simulink model "Electron_Rocket_test_failed"  (R2023a)
settings: Solver=ode45  StartTime=0.0  StopTime=5000  RelTol=1e-6
undefined symbols (not defined in the file or in its folder): Earth, WGS84
libraries: simulink x3, aerolibadyn x1, aerolibatmos2 x1, slpidlib x1, simulink_extras x1, aerolib6dof2 x1
settings Model: Creator=User  LastModifiedBy=User

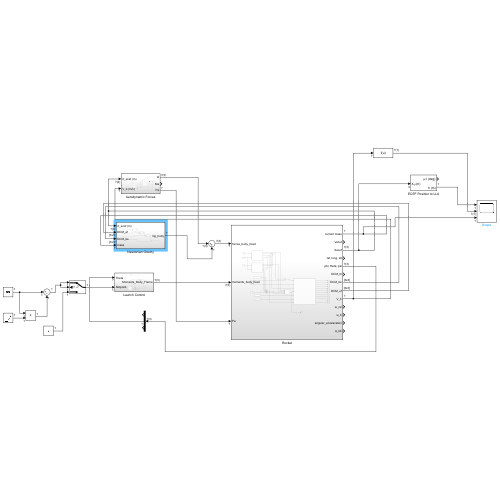
[thumbnail: Simulink's stored preview of the top-level diagram]
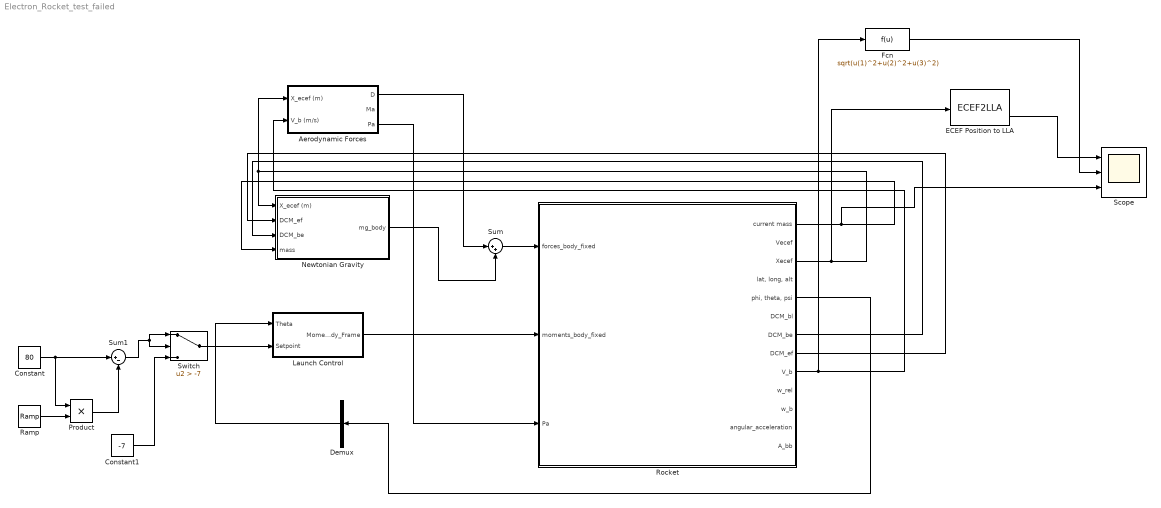
== system Electron_Rocket_test_failed ==
  Aerodynamic Forces : Subsystem
  Constant : Constant  Value=80
  Constant1 : Constant  Value=-7
  Demux : Demux  Outputs=3
  ECEF Position to LLA : ECEF2LLA
  Fcn : Fcn  Expr=sqrt(u(1)^2+u(2)^2+u(3)^2)
  Launch Control : Subsystem
  Newtonian Gravity : Subsystem
  Product : Product
  Ramp : simulink/Sources/Ramp  slope=0.0085  start=15  InitialOutput=0
  Rocket : Subsystem
  Scope : Scope  NumInputPorts=3
  Sum : Sum  Inputs=|++
  Sum1 : Sum  Inputs=|+-
  Switch : Switch  Criteria=u2 > Threshold  Threshold=-7  SaturateOnIntegerOverflow=off  InputSameDT=off
  wires:
  Rocket/3(Xecef) -> ECEF Position to LLA/1, Aerodynamic Forces/1(X_ecef (m)), Newtonian Gravity/1(X_ecef (m))
  Rocket/9(V_b) -> Fcn/1, Aerodynamic Forces/2(V_b (m/s))
  Rocket/1(current mass) -> Scope/3, Newtonian Gravity/4(mass)
  Rocket/7(DCM_be) -> Newtonian Gravity/3(DCM_be)
  Rocket/8(DCM_ef) -> Newtonian Gravity/2(DCM_ef)
  Aerodynamic Forces/1(D) -> Sum/1
  Newtonian Gravity/1(mg_body) -> Sum/2
  Sum/1 -> Rocket/1(forces_body_fixed)
  Aerodynamic Forces/3(Pa) -> Rocket/3(Pa)
  Launch Control/1(Moments_Body_Frame) -> Rocket/2(moments_body_fixed)
  Rocket/5("phi, theta, psi") -> Demux/1
  Demux/2 -> Launch Control/1(Theta)
  Constant/1 -> Sum1/1, Product/1
  Ramp/1 -> Product/2
  Sum1/1 -> Switch/1, Switch/2
  Switch/1 -> Launch Control/2(Setpoint)
  Constant1/1 -> Switch/3
  Product/1 -> Sum1/2
  ECEF Position to LLA/2 -> Scope/1
  Fcn/1 -> Scope/2

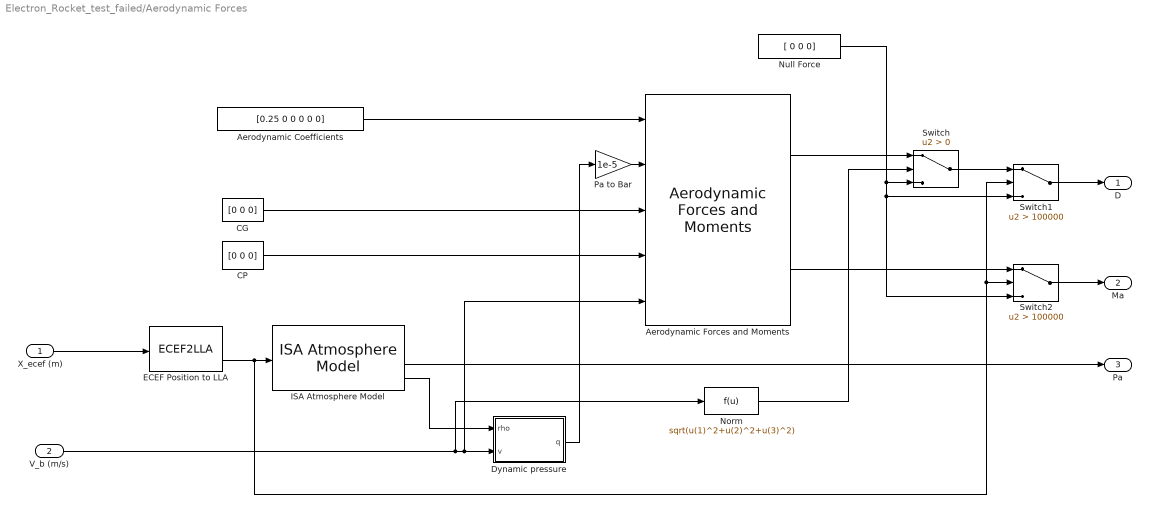
== system Electron_Rocket_test_failed/Aerodynamic Forces ==
  X_ecef (m) : Inport
  V_b (m/s) : Inport  Port=2
  "Aerodynamic Forces and Moments " : aerolibadyn/Aerodynamic Forces and Moments   inputAxes=Wind  outputForceAxes=Body  outputMomentAxes=Body  S=0.78  b=1  cbar=17
  Aerodynamic Coefficients : Constant  Value=[0.25 0 0 0 0 0]
  CG : Constant  Value=[0 0 0]
  CP : Constant  Value=[0 0 0]
  Dynamic pressure : MATLAB Function  TreatAsAtomicUnit=on
  ECEF Position to LLA : ECEF2LLA
  ISA Atmosphere Model : aerolibatmos2/ISA Atmosphere Model  custom=off  g=9.80665  gamma=1.4  R=287.0531  L=0.0065  h_trop=11000  h_strat=20000  rho0=1.225  P0=101325  T0=288.15  h0=0
  Norm : Fcn  Expr=sqrt(u(1)^2+u(2)^2+u(3)^2)
  Null Force : Constant  Value=[ 0 0 0]
  Pa to Bar : Gain  Gain=1e-5
  Switch : Switch  Criteria=u2 > Threshold  SaturateOnIntegerOverflow=off  InputSameDT=off
  Switch1 : Switch  Criteria=u2 > Threshold  Threshold=100000  SaturateOnIntegerOverflow=off  InputSameDT=off
  Switch2 : Switch  Criteria=u2 > Threshold  Threshold=100000  SaturateOnIntegerOverflow=off  InputSameDT=off
  D : Outport
  Ma : Outport  Port=2
  Pa : Outport  Port=3
  wires:
  X_ecef (m)/1 -> ECEF Position to LLA/1
  ISA Atmosphere Model/3 -> Pa/1
  CP/1 -> "Aerodynamic Forces and Moments "/4
  CG/1 -> "Aerodynamic Forces and Moments "/3
  V_b (m/s)/1 -> Norm/1, "Aerodynamic Forces and Moments "/5, Dynamic pressure/2(v)
  ISA Atmosphere Model/4 -> Dynamic pressure/1(rho)
  Dynamic pressure/1(q) -> Pa to Bar/1
  Pa to Bar/1 -> "Aerodynamic Forces and Moments "/2
  Aerodynamic Coefficients/1 -> "Aerodynamic Forces and Moments "/1
  Norm/1 -> Switch/2
  "Aerodynamic Forces and Moments "/1 -> Switch/1
  Null Force/1 -> Switch/3, Switch2/3, Switch1/3
  Switch/1 -> Switch1/1
  Switch1/1 -> D/1
  ECEF Position to LLA/2 -> Switch2/2, Switch1/2, ISA Atmosphere Model/1
  "Aerodynamic Forces and Moments "/2 -> Switch2/1
  Switch2/1 -> Ma/1

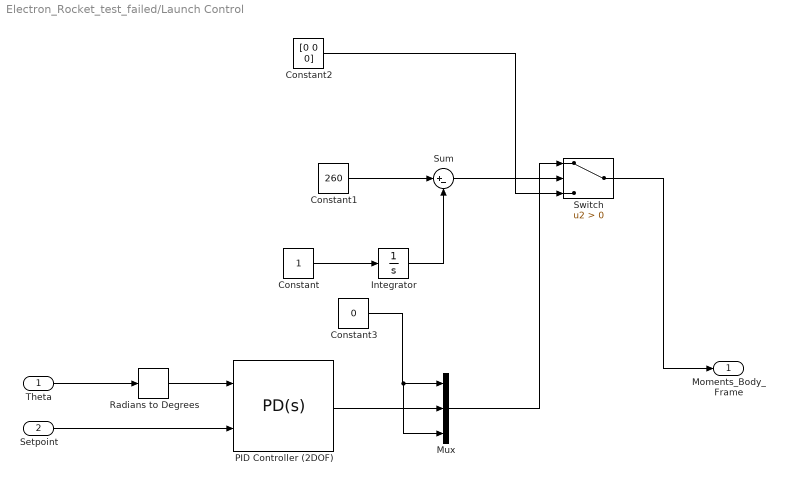
== system Electron_Rocket_test_failed/Launch Control ==
  Theta : Inport
  Setpoint : Inport  Port=2
  Constant : Constant
  Constant1 : Constant  Value=260
  Constant2 : Constant  Value=[0 0 0]
  Constant3 : Constant  Value=0
  Integrator : Integrator
  Mux : Mux  Inputs=3
  PID Controller (2DOF) : slpidlib/PID Controller (2DOF)  Controller=PD  Form=Parallel  TimeDomain=Continuous-time  UseExternalTs=off  SampleTime=-1  IntegratorMethod=Forward Euler  FilterMethod=Forward Euler  ControllerParametersSource=internal  P=0.01  I=0  UseKiTs=off  D=0.01  N=100  UseFilter=on  b=1  c=1  TunerSelectOption=Transfer Function Based (PID Tuner App)  InitialConditionSource=internal  InitialConditionForIntegrator=0  InitialConditionForFilter=0  DifferentiatorICPrevScaledInput=0  ExternalReset=none  TrackingMode=off  Kt=1  LimitOutput=off  SatLimitsSource=internal  UpperSaturationLimit=inf  LowerSaturationLimit=-inf  LinearizeAsGain=on  AntiWindupMode=none  Kb=1  LimitIntegrator=off  UpperIntegratorSaturationLimit=inf  LowerIntegratorSaturationLimit=-inf  POutMin=[]  POutMax=[]  IOutMin=[]  IOutMax=[]  DOutMin=[]  DOutMax=[]  NOutMin=[]  NOutMax=[]  bOutMin=[]  bOutMax=[]  cOutMin=[]  cOutMax=[]  SumOutMin=[]  SumOutMax=[]  SaturationOutMin=[]  SaturationOutMax=[]  PParamMin=[]  PParamMax=[]  IParamMin=[]  IParamMax=[]  DParamMin=[]  DParamMax=[]  NParamMin=[]  NParamMax=[]  bParamMin=[]  bParamMax=[]  cParamMin=[]  cParamMax=[]  KbParamMin=[]  KbParamMax=[]  KtParamMin=[]  KtParamMax=[]  KbOutMin=[]  KbOutMax=[]  KtOutMin=[]  KtOutMax=[]  IntegratorOutMin=[]  IntegratorOutMax=[]  FilterOutMin=[]  FilterOutMax=[]  SumI1OutMin=[]  SumI1OutMax=[]  SumI2OutMin=[]  SumI2OutMax=[]  SumI3OutMin=[]  SumI3OutMax=[]  SumI4OutMin=[]  SumI4OutMax=[]  SumDOutMin=[]  SumDOutMax=[]  Sum1OutMin=[]  Sum1OutMax=[]  Sum2OutMin=[]  Sum2OutMax=[]  Sum3OutMin=[]  Sum3OutMax=[]  DifferentiatorOutMin=[]  DifferentiatorOutMax=[]  FilterDiffOutCoefMin=[]  FilterDiffOutCoefMax=[]  ReciprocalOutMin=[]  ReciprocalOutMax=[]  SumDenOutMin=[]  SumDenOutMax=[]  SumNumOutMin=[]  SumNumOutMax=[]  DivideOutMin=[]  DivideOutMax=[]  UdiffTsProdOutMin=[]  UdiffTsProdOutMax=[]  NTsProdOutMin=[]  NTsProdOutMax=[]  UintegralTsProdOutMin=[]  UintegralTsProdOutMax=[]  UngainTsProdOutMin=[]  UngainTsProdOutMax=[]  ClampingZeroOutDataTypeStr=Inherit: Inherit via back propagation  ClampingZeroOutMin=[]  ClampingZeroOutMax=[]  FilterDenConstantOutDataTypeStr=Inherit: Inherit via back propagation  FilterDenConstantOutMin=[]  FilterDenConstantOutMax=[]  PCopyOutDataTypeStr=Inherit: Inherit via back propagation  PCopyOutMin=[]  PCopyOutMax=[]  NCopyOutDataTypeStr=Inherit: Inherit via back propagation  NCopyOutMin=[]  NCopyOutMax=[]  IntegratorContinuousStateAttributes=''  IntegratorStateMustResolveToSignalObject=off  IntegratorRTWStateStorageClass=Auto  FilterContinuousStateAttributes=''  FilterStateMustResolveToSignalObject=off  FilterRTWStateStorageClass=Auto  ParallelPVariant=InternalParameters  IdealPVariant=Disabled  IVariant=Disabled  DVariant=InternalParameters  bVariant=InternalParameters  cVariant=InternalParameters  IntegratorVariant=Disabled  SatVariant=Disabled  AWVariant=Disabled  PCopyVariant=Disabled  TRVariant=Disabled  FdbkBlocksVariant=Forward  IdealPFdbkVariant=Disabled  SatFdbkVariant=Disabled  DerivativeFilterVariant=ContFilter  NVariant=InternalParameters  NCopyVariant=Disabled  FilterICVariant=InternalICsFilter  IntegratorICVariant=Disabled  ExternalResetVariant=Disabled  TRSumVariant=Passthrough  SumFdbkVariant=Disabled  SumVariant=Sum_PD  TsampFilterVariant=InternalTs  TsampNgainVariant=Passthrough  TsampIntegralVariant=Disabled_SignalSpec  ExternalSaturationOutDataTypeStr=Inherit: Same as second input
  Radians to Degrees : simulink_extras/Transformations/Radians to Degrees
  Sum : Sum  Inputs=|+-
  Switch : Switch  Criteria=u2 > Threshold  SaturateOnIntegerOverflow=off  InputSameDT=off
  Moments_Body_Frame : Outport
  wires:
  Theta/1 -> Radians to Degrees/1
  Radians to Degrees/1 -> PID Controller (2DOF)/1
  Constant/1 -> Integrator/1
  Constant1/1 -> Sum/1
  Sum/1 -> Switch/2
  Switch/1 -> Moments_Body_Frame/1
  Constant2/1 -> Switch/3
  Constant3/1 -> Mux/3, Mux/1
  Integrator/1 -> Sum/2
  PID Controller (2DOF)/1 -> Mux/2
  Mux/1 -> Switch/1
  Setpoint/1 -> PID Controller (2DOF)/2

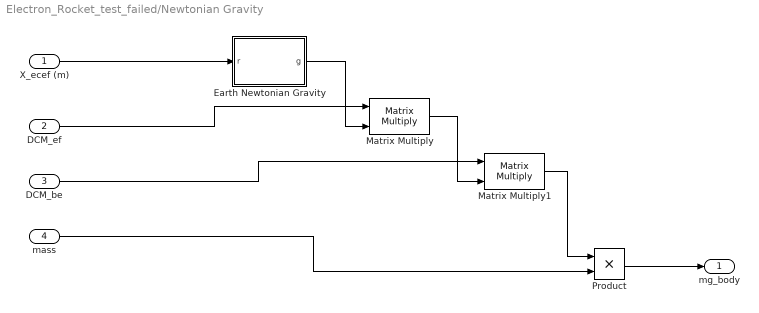
== system Electron_Rocket_test_failed/Newtonian Gravity ==
  X_ecef (m) : Inport
  DCM_ef : Inport  Port=2
  DCM_be : Inport  Port=3
  mass : Inport  Port=4
  Earth Newtonian Gravity : MATLAB Function  TreatAsAtomicUnit=on
  Matrix Multiply : Product  Multiplication=Matrix(*)
  Matrix Multiply1 : Product  Multiplication=Matrix(*)
  Product : Product
  mg_body : Outport
  wires:
  X_ecef (m)/1 -> Earth Newtonian Gravity/1(r)
  Matrix Multiply1/1 -> Product/1
  Product/1 -> mg_body/1
  mass/1 -> Product/2
  DCM_ef/1 -> Matrix Multiply/1
  Earth Newtonian Gravity/1(g) -> Matrix Multiply/2
  Matrix Multiply/1 -> Matrix Multiply1/2
  DCM_be/1 -> Matrix Multiply1/1

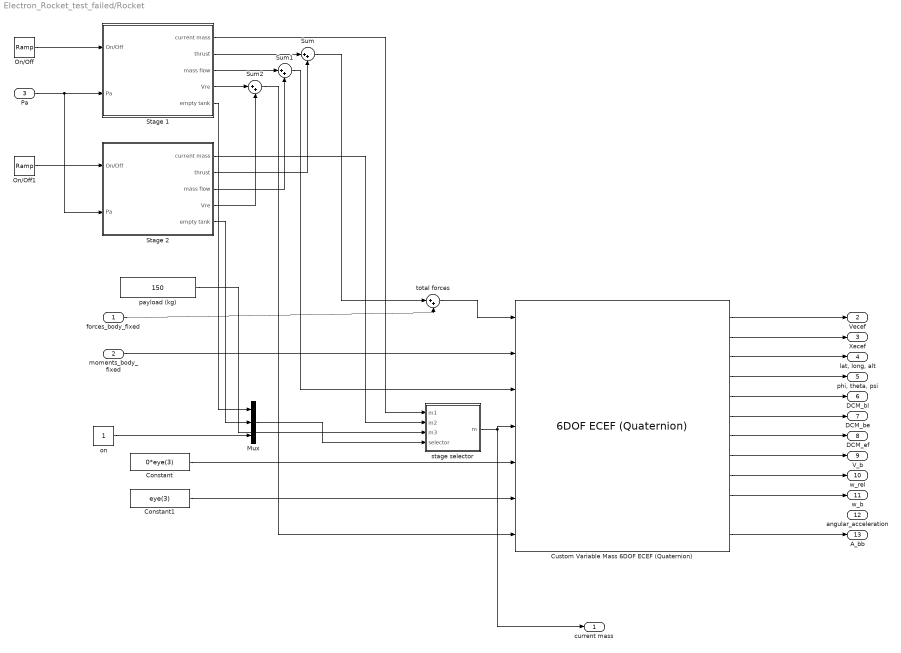
== system Electron_Rocket_test_failed/Rocket ==
  forces_body_fixed : Inport
  moments_body_fixed : Inport  Port=2
  Pa : Inport  Port=3
  Constant : Constant  Value=0*eye(3)
  Constant1 : Constant  Value=eye(3)
  Custom Variable Mass 6DOF ECEF (Quaternion) : aerolib6dof2/6DOF ECEF (Quaternion)  units=Metric (MKS)  mtype=Custom Variable  xg_0=[35.31 -117.48 2000]  Vm_0=[0 0 0]  eul_0=[0 90 0]  pm_0=[0 0 0]  mass_0=1.0  mass_e=0.5  mass_f=2.0  inertia=eye(3)  inertia_e=eye(3)  inertia_f=2*eye(3)  vre_flag=on  abi_flag=off  ptype=Earth (WGS84)  R=6378137  F=1/298.257223563  w_E=7292115e-11  angle_in=Internal  LG0=0  quat_statename=''  pm_statename=''  Vm_statename=''  posECEF_statename=''  posECI_statename=''  LG_statename=''  mass_statename=''
      settings: LibrarySourceBlock=|
      | aerolib6dof2/Custom Variable Mass 6DOF
      | ECEF (Quaternion)
  Mux : Mux  Inputs=3
  On/Off : simulink/Sources/Ramp  slope=1  start=0  InitialOutput=0
  On/Off1 : simulink/Sources/Ramp  slope=1  start=129  InitialOutput=0
  Stage 1 : Subsystem
  Stage 2 : Subsystem
  Sum : Sum  Inputs=|++
  Sum1 : Sum  Inputs=|++
  Sum2 : Sum  Inputs=|++
  on : Constant
  payload (kg) : Constant  Value=150
  stage selector : MATLAB Function  TreatAsAtomicUnit=on
  total forces : Sum  Inputs=|++
  current mass : Outport
  Vecef : Outport  Port=2
  Xecef : Outport  Port=3
  "lat, long, alt" : Outport  Port=4
  "phi, theta, psi" : Outport  Port=5
  DCM_bl : Outport  Port=6
  DCM_be : Outport  Port=7
  DCM_ef : Outport  Port=8
  V_b : Outport  Port=9
  w_rel : Outport  Port=10
  w_b : Outport  Port=11
  angular_acceleration : Outport  Port=12
  A_bb : Outport  Port=13
  wires:
  total forces/1 -> Custom Variable Mass 6DOF ECEF (Quaternion)/1
  Pa/1 -> Stage 2/2(Pa), Stage 1/2(Pa)
  stage selector/1(m) -> Custom Variable Mass 6DOF ECEF (Quaternion)/4, current mass/1
  forces_body_fixed/1 -> total forces/2
  Custom Variable Mass 6DOF ECEF (Quaternion)/10 -> w_b/1
  Mux/1 -> stage selector/4(selector)
  Custom Variable Mass 6DOF ECEF (Quaternion)/7 -> DCM_ef/1
  Custom Variable Mass 6DOF ECEF (Quaternion)/12 -> A_bb/1
  Custom Variable Mass 6DOF ECEF (Quaternion)/9 -> w_rel/1
  Custom Variable Mass 6DOF ECEF (Quaternion)/5 -> DCM_bl/1
  Custom Variable Mass 6DOF ECEF (Quaternion)/4 -> "phi, theta, psi"/1
  On/Off/1 -> Stage 1/1(On/Off)
  Constant/1 -> Custom Variable Mass 6DOF ECEF (Quaternion)/5
  moments_body_fixed/1 -> Custom Variable Mass 6DOF ECEF (Quaternion)/2
  Custom Variable Mass 6DOF ECEF (Quaternion)/2 -> Xecef/1
  Custom Variable Mass 6DOF ECEF (Quaternion)/1 -> Vecef/1
  Constant1/1 -> Custom Variable Mass 6DOF ECEF (Quaternion)/6
  Custom Variable Mass 6DOF ECEF (Quaternion)/8 -> V_b/1
  Custom Variable Mass 6DOF ECEF (Quaternion)/6 -> DCM_be/1
  Custom Variable Mass 6DOF ECEF (Quaternion)/3 -> "lat, long, alt"/1
  Stage 1/2(thrust) -> Sum/1
  Stage 2/2(thrust) -> Sum/2
  Sum/1 -> total forces/1
  Stage 1/3(mass flow) -> Sum1/1
  Stage 2/3(mass flow) -> Sum1/2
  Sum1/1 -> Custom Variable Mass 6DOF ECEF (Quaternion)/3
  Stage 1/4(Vre) -> Sum2/1
  Stage 2/4(Vre) -> Sum2/2
  Sum2/1 -> Custom Variable Mass 6DOF ECEF (Quaternion)/7
  Stage 1/1(current mass) -> stage selector/1(m1)
  Stage 2/1(current mass) -> stage selector/2(m2)
  payload (kg)/1 -> stage selector/3(m3)
  Stage 1/5(empty tank) -> Mux/1
  Stage 2/5(empty tank) -> Mux/2
  on/1 -> Mux/3
  On/Off1/1 -> Stage 2/1(On/Off)

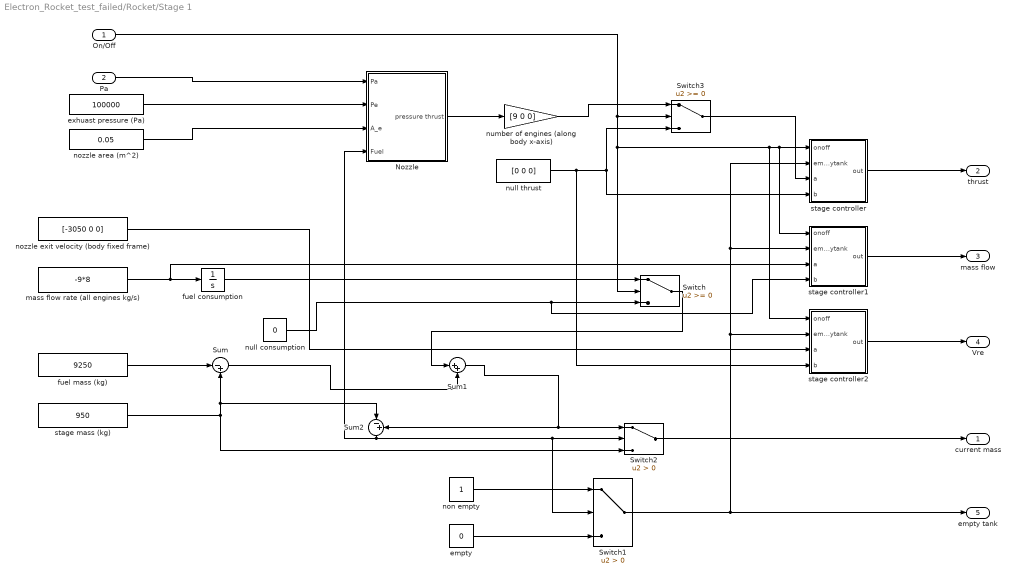
== system Electron_Rocket_test_failed/Rocket/Stage 1 ==
  On/Off : Inport
  Pa : Inport  Port=2
  Nozzle : Subsystem
  Sum : Sum  Inputs=|-+
  Sum1 : Sum  Inputs=|++
  Sum2 : Sum  Inputs=|-+
  Switch : Switch  SaturateOnIntegerOverflow=off  InputSameDT=off
  Switch1 : Switch  Criteria=u2 > Threshold  SaturateOnIntegerOverflow=off  InputSameDT=off
  Switch2 : Switch  Criteria=u2 > Threshold  SaturateOnIntegerOverflow=off  InputSameDT=off
  Switch3 : Switch  SaturateOnIntegerOverflow=off  InputSameDT=off
  empty : Constant  Value=0
  exhuast pressure (Pa) : Constant  Value=100000
  fuel consumption : Integrator
  fuel mass (kg) : Constant  Value=9250
  mass flow rate (all engines kg/s) : Constant  Value=-9*8
  non empty : Constant
  nozzle area (m^2) : Constant  Value=0.05
  nozzle exit velocity (body fixed frame) : Constant  Value=[-3050 0 0]
  null consumption : Constant  Value=0
  null thrust : Constant  Value=[0 0 0]
  number of engines (along body x-axis) : Gain  Gain=[9 0 0]
  stage controller : MATLAB Function  TreatAsAtomicUnit=on
  stage controller1 : MATLAB Function  TreatAsAtomicUnit=on
  stage controller2 : MATLAB Function  TreatAsAtomicUnit=on
  stage mass (kg) : Constant  Value=950
  current mass : Outport
  thrust : Outport  Port=2
  mass flow : Outport  Port=3
  Vre : Outport  Port=4
  empty tank : Outport  Port=5
  wires:
  nozzle area (m^2)/1 -> Nozzle/3(A_e)
  exhuast pressure (Pa)/1 -> Nozzle/2(Pe)
  Pa/1 -> Nozzle/1(Pa)
  Nozzle/1(pressure thrust) -> number of engines (along body x-axis)/1
  fuel mass (kg)/1 -> Sum/1
  stage mass (kg)/1 -> Switch2/3, Sum2/1, Sum/2
  Sum/1 -> Sum1/2
  mass flow rate (all engines kg/s)/1 -> stage controller1/3(a), fuel consumption/1
  fuel consumption/1 -> Switch/1
  null consumption/1 -> stage controller1/4(b), Switch/3
  On/Off/1 -> Switch3/2, stage controller2/1(onoff), stage controller1/1(onoff), stage controller/1(onoff), Switch/2
  Switch/1 -> Sum1/1
  Sum1/1 -> Switch2/1, Sum2/2
  Switch1/1 -> stage controller2/2(emptytank), stage controller1/2(emptytank), stage controller/2(emptytank), empty tank/1
  non empty/1 -> Switch1/1
  empty/1 -> Switch1/3
  Sum2/1 -> Switch1/2, Switch2/2, Nozzle/4(Fuel)
  stage controller/1(out) -> thrust/1
  stage controller1/1(out) -> mass flow/1
  stage controller2/1(out) -> Vre/1
  Switch2/1 -> current mass/1
  number of engines (along body x-axis)/1 -> Switch3/1
  Switch3/1 -> stage controller/3(a)
  null thrust/1 -> stage controller2/4(b), Switch3/3, stage controller/4(b)
  nozzle exit velocity (body fixed frame)/1 -> stage controller2/3(a)

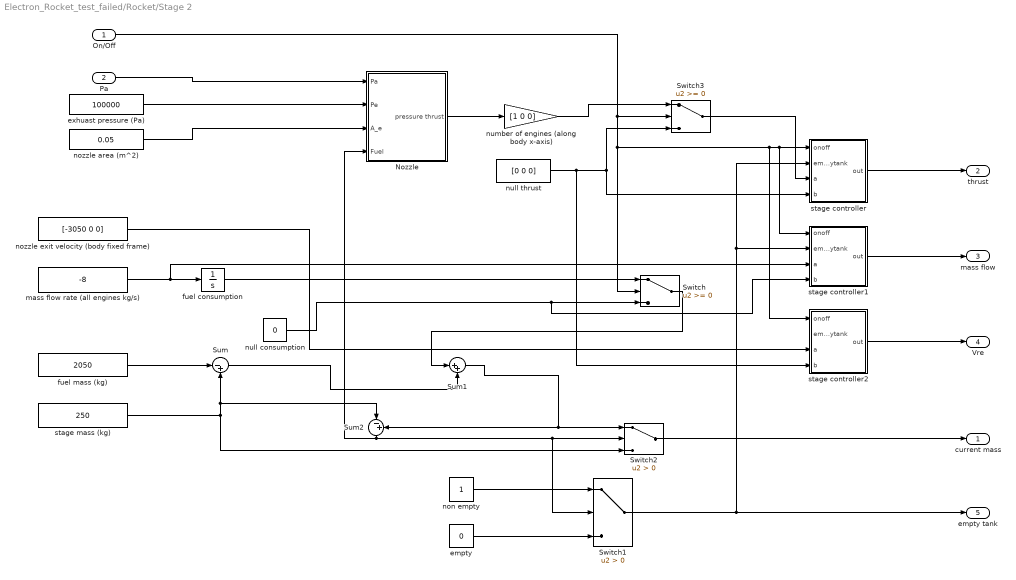
== system Electron_Rocket_test_failed/Rocket/Stage 2 ==
  On/Off : Inport
  Pa : Inport  Port=2
  Nozzle : Subsystem
  Sum : Sum  Inputs=|-+
  Sum1 : Sum  Inputs=|++
  Sum2 : Sum  Inputs=|-+
  Switch : Switch  SaturateOnIntegerOverflow=off  InputSameDT=off
  Switch1 : Switch  Criteria=u2 > Threshold  SaturateOnIntegerOverflow=off  InputSameDT=off
  Switch2 : Switch  Criteria=u2 > Threshold  SaturateOnIntegerOverflow=off  InputSameDT=off
  Switch3 : Switch  SaturateOnIntegerOverflow=off  InputSameDT=off
  empty : Constant  Value=0
  exhuast pressure (Pa) : Constant  Value=100000
  fuel consumption : Integrator
  fuel mass (kg) : Constant  Value=2050
  mass flow rate (all engines kg/s) : Constant  Value=-8
  non empty : Constant
  nozzle area (m^2) : Constant  Value=0.05
  nozzle exit velocity (body fixed frame) : Constant  Value=[-3050 0 0]
  null consumption : Constant  Value=0
  null thrust : Constant  Value=[0 0 0]
  number of engines (along body x-axis) : Gain  Gain=[1 0 0]
  stage controller : MATLAB Function  TreatAsAtomicUnit=on
  stage controller1 : MATLAB Function  TreatAsAtomicUnit=on
  stage controller2 : MATLAB Function  TreatAsAtomicUnit=on
  stage mass (kg) : Constant  Value=250
  current mass : Outport
  thrust : Outport  Port=2
  mass flow : Outport  Port=3
  Vre : Outport  Port=4
  empty tank : Outport  Port=5
  wires:
  nozzle area (m^2)/1 -> Nozzle/3(A_e)
  exhuast pressure (Pa)/1 -> Nozzle/2(Pe)
  Pa/1 -> Nozzle/1(Pa)
  Nozzle/1(pressure thrust) -> number of engines (along body x-axis)/1
  fuel mass (kg)/1 -> Sum/1
  stage mass (kg)/1 -> Switch2/3, Sum2/1, Sum/2
  Sum/1 -> Sum1/2
  mass flow rate (all engines kg/s)/1 -> stage controller1/3(a), fuel consumption/1
  fuel consumption/1 -> Switch/1
  null consumption/1 -> stage controller1/4(b), Switch/3
  On/Off/1 -> Switch3/2, stage controller2/1(onoff), stage controller1/1(onoff), stage controller/1(onoff), Switch/2
  Switch/1 -> Sum1/1
  Sum1/1 -> Switch2/1, Sum2/2
  Switch1/1 -> stage controller1/2(emptytank), stage controller/2(emptytank), empty tank/1
  non empty/1 -> Switch1/1
  empty/1 -> Switch1/3
  Sum2/1 -> Switch1/2, Switch2/2, Nozzle/4(Fuel)
  stage controller/1(out) -> thrust/1
  stage controller1/1(out) -> mass flow/1
  stage controller2/1(out) -> Vre/1
  Switch2/1 -> current mass/1
  number of engines (along body x-axis)/1 -> Switch3/1
  Switch3/1 -> stage controller/3(a)
  null thrust/1 -> stage controller2/4(b), Switch3/3, stage controller/4(b)
  nozzle exit velocity (body fixed frame)/1 -> stage controller2/3(a)

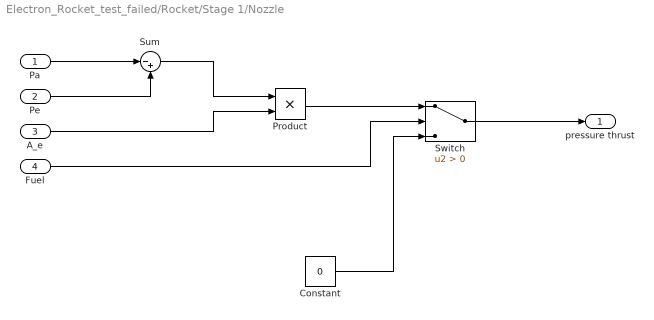
== system Electron_Rocket_test_failed/Rocket/Stage 1/Nozzle ==
  Pa : Inport
  Pe : Inport  Port=2
  A_e : Inport  Port=3
  Fuel : Inport  Port=4
  Constant : Constant  Value=0
  Product : Product
  Sum : Sum  Inputs=|-+
  Switch : Switch  Criteria=u2 > Threshold  SaturateOnIntegerOverflow=off  InputSameDT=off
  pressure thrust : Outport
  wires:
  Pe/1 -> Sum/2
  Pa/1 -> Sum/1
  Sum/1 -> Product/1
  A_e/1 -> Product/2
  Product/1 -> Switch/1
  Fuel/1 -> Switch/2
  Constant/1 -> Switch/3
  Switch/1 -> pressure thrust/1

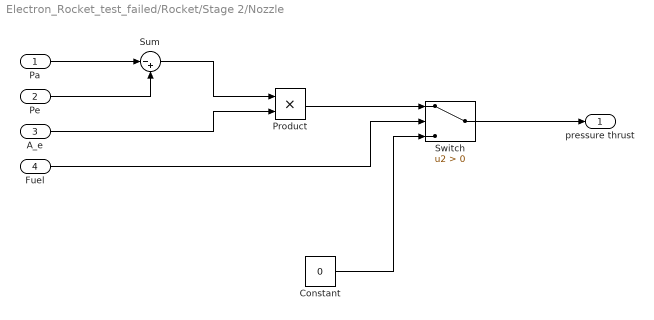
== system Electron_Rocket_test_failed/Rocket/Stage 2/Nozzle ==
  Pa : Inport
  Pe : Inport  Port=2
  A_e : Inport  Port=3
  Fuel : Inport  Port=4
  Constant : Constant  Value=0
  Product : Product
  Sum : Sum  Inputs=|-+
  Switch : Switch  Criteria=u2 > Threshold  SaturateOnIntegerOverflow=off  InputSameDT=off
  pressure thrust : Outport
  wires:
  Pe/1 -> Sum/2
  Pa/1 -> Sum/1
  Sum/1 -> Product/1
  A_e/1 -> Product/2
  Product/1 -> Switch/1
  Fuel/1 -> Switch/2
  Constant/1 -> Switch/3
  Switch/1 -> pressure thrust/1

== matlab function Electron_Rocket_test_failed/Aerodynamic Forces/Dynamic pressure ==
  data: rho input; q output; v input
function q = fcn(rho, v)
q = (1/2)*rho*dot(v,v);

== matlab function Electron_Rocket_test_failed/Newtonian Gravity/Earth Newtonian Gravity ==
  data: r input; g output
function g = fcn(r)
mu = 3.956004415e14;
g = -(mu/norm(r)^3).*(r);

== matlab function Electron_Rocket_test_failed/Rocket/Stage 2/stage controller ==
  data: onoff input; out output; emptytank input; a input; b input
function out = fcn(onoff, emptytank, a, b)
%#codegen
if onoff >= 1 && emptytank== 1
    out = a;
else
    out = b;
end

== matlab function Electron_Rocket_test_failed/Rocket/Stage 2/stage controller1 ==
  data: onoff input; out output; emptytank input; a input; b input
function out = fcn(onoff, emptytank, a, b)
%#codegen
if onoff >= 1 && emptytank == 1
    out = a;
else
    out = b;
end

== matlab function Electron_Rocket_test_failed/Rocket/Stage 1/stage controller ==
  data: onoff input; out output; emptytank input; a input; b input
function out = fcn(onoff, emptytank, a, b)
%#codegen
if onoff >= 1 && emptytank == 1
    out = a;
else
    out = b;
end

== matlab function Electron_Rocket_test_failed/Rocket/Stage 1/stage controller1 ==
  data: onoff input; out output; emptytank input; a input; b input
function out = fcn(onoff, emptytank, a, b)
%#codegen
if onoff >= 1 && emptytank == 1
    out = a;
else
    out = b;
end

== matlab function Electron_Rocket_test_failed/Rocket/Stage 1/stage controller2 ==
  data: onoff input; out output; emptytank input; a input; b input
function out = fcn(onoff, emptytank, a, b)
%#codegen
if onoff >= 1 && emptytank == 1
    out = a;
else
    out = b;
end

== matlab function Electron_Rocket_test_failed/Rocket/stage selector ==
  data: m1 input; m output; m2 input; m3 input; selector input
function m = fcn(m1, m2, m3, selector)
m = 0;
if selector(1) == 1
    m = m + m1;
end
if selector(2) == 1
    m = m + m2;
end
if selector(3) == 1
    m = m + m3;
end

== matlab function Electron_Rocket_test_failed/Rocket/Stage 2/stage controller2 ==
  data: onoff input; out output; emptytank input; a input; b input
function out = fcn(onoff, emptytank, a, b)
%#codegen
if onoff >= 1 && emptytank == 1
    out = a;
else
    out = b;
end
